simulink model "envelope_detection_hilbert"  (R2021b)
settings: Solver=FixedStepDiscrete  StartTime=0.0  StopTime=0.01  FixedStep=5e-07  RelTol=1e-3
settings Model: Creator=caccolillo  LastModifiedBy=caccolillo

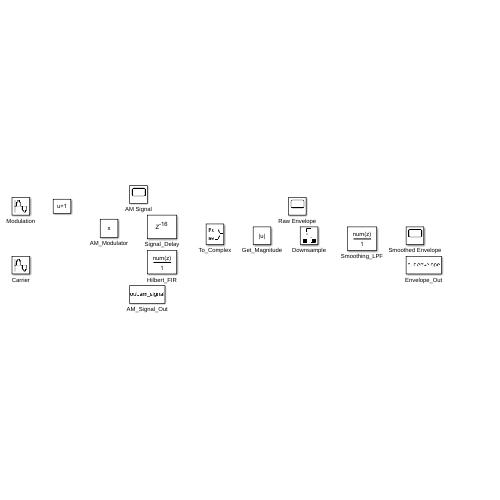
[thumbnail: Simulink's stored preview of the top-level diagram]
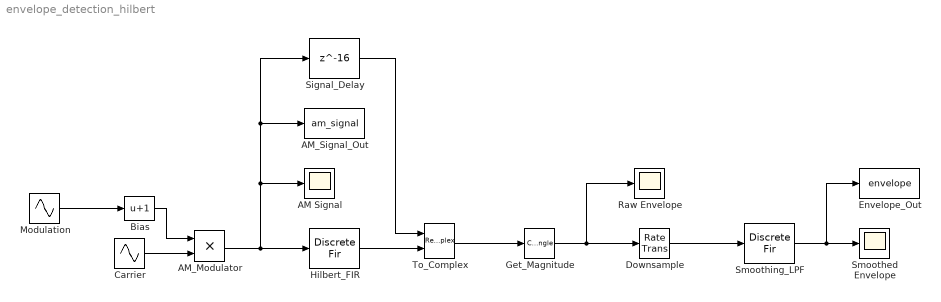
== system envelope_detection_hilbert ==
  AM Signal : Scope
  AM_Modulator : Product
  AM_Signal_Out : ToWorkspace  VariableName=am_signal  SampleTime=-1
  Bias : Bias  Bias=1
  Carrier : Sin  Frequency=500000  SampleTime=5e-07
  Downsample : RateTransition  OutPortSampleTime=1e-05
  Envelope_Out : ToWorkspace  VariableName=envelope  SampleTime=-1
  Get_Magnitude : ComplexToMagnitudeAngle  Output=Magnitude
  Hilbert_FIR : DiscreteFir  Coefficients=[-0.00308389580700725 -0.00115633221688013 -0.00597083169399809 -0.0033653501813807 -0.0113702945955279 -0.00756834405893307 -0.0196285156439845 -0.0149781861053033 -0.0321135512664649 -0.0278947866237693 -0.0520566925518648 -0.052256610273355 -0.0903025345724302 -0.112588487998692 -0.217003149479529 -0.626555340283115 0.626555340283115 0.217003149479529 0.112588487998692 0.0903025345724302 0.052256610273355 0.0520566925518648 0.0278947866237693 0.0321135512664649 0.0149781861053033 0.0196285156439845 0.00756834405893307 0.0113702945955279 0.0033653501813807 0.00597083169399809 0.00115633221688013 0.00308389580700725]
  Modulation : Sin  Amplitude=0.8  Frequency=50  SampleTime=5e-07
  Raw Envelope : Scope
  Signal_Delay : Delay  DelayLength=16
  Smoothed Envelope : Scope
  Smoothing_LPF : DiscreteFir  Coefficients=[0.00101602337453036 0.00105219577870945 0.00105485683106792 0.000952665359447147 0.000639612341797336 -6.52666866268383e-19 -0.00105692963887472 -0.00255869545799197 -0.00443506164976659 -0.006494969918075 -0.00842139827326761 -0.00978815640308439 -0.0100992191521871 -0.00884737843452352 -0.00558538708219877 2.65242471953122e-18 0.00802209630348964 0.0183472205804422 0.0305752786568395 0.0440532963650553 0.0579227189698704 0.0711964425915403 0.0828570731115069 0.0919645189858877 0.0977592659894717 0.0997478615406278 0.0977592659894717 0.0919645189858877 0.0828570731115069 0.0711964425915403 0.0579227189698704 0.0440532963650553 0.0305752786568395 0.0183472205804422 0.00802209630348964 2.65242471953122e-18 -0.00558538708219877 -0.00884737843452352 -0.0100992191521871 -0.00978815640308439 -0.00842139827326761 -0.006494969918075 -0.00443506164976659 -0.00255869545799197 -0.00105692963887472 -6.52666866268383e-19 0.000639612341797336 0.000952665359447147 0.00105485683106792 0.00105219577870945 0.00101602337453036]
  To_Complex : RealImagToComplex
  wires:
  Smoothing_LPF/1 -> Smoothed Envelope/1, Envelope_Out/1
  Modulation/1 -> Bias/1
  To_Complex/1 -> Get_Magnitude/1
  Get_Magnitude/1 -> Raw Envelope/1, Downsample/1
  Downsample/1 -> Smoothing_LPF/1
  AM_Modulator/1 -> Signal_Delay/1, AM_Signal_Out/1, AM Signal/1, Hilbert_FIR/1
  Hilbert_FIR/1 -> To_Complex/2
  Carrier/1 -> AM_Modulator/2
  Signal_Delay/1 -> To_Complex/1
  Bias/1 -> AM_Modulator/1
